simulink model "spike_detection"  (R2020a)
settings: Solver=FixedStepDiscrete  StartTime=0.0  StopTime=840000  RelTol=1e-3
libraries: hdlsllib x8, simulink x4
settings Model: FPTRunName=FPA_Reference  PacingRate=40  Creator=BuccelliLab  LastModifiedBy=diflo
settings SolverCC: AutoInsertRateTranBlk=on  MinimalZcImpactIntegration=on
settings DataIOCC: LimitDataPoints=on  SaveOutput=off  SaveTime=off  ReturnWorkspaceOutputs=off
settings OptimizationCC: BlockReduction=off  ConditionallyExecuteInputs=off  DefaultParameterBehavior=Inlined  LifeSpan=inf
settings DebuggingCC: SignalRangeChecking=warning  ReadBeforeWriteMsg=DisableAll  WriteAfterWriteMsg=DisableAll  WriteAfterReadMsg=DisableAll  AlgebraicLoopMsg=error  MultiTaskDSMMsg=none  SingleTaskRateTransMsg=error  ParameterDowncastMsg=warning  ParameterOverflowMsg=warning  AllowSymbolicDim=off  StrictBusMsg=ErrorOnBusTreatedAsVector  SFUnexpectedBacktrackingDiag=warning  SFNoUnconditionalDefaultTransitionDiag=warning  SFExecutionAtInitializationDiag=none  ArithmeticOperatorsInVariantConditions=warning
settings HardwareCC: ProdBitPerPointer=32  ProdBitPerSizeT=32  ProdBitPerPtrDiffT=32  ProdLargestAtomicFloat=None  ProdIntDivRoundTo=Undefined  ProdEndianess=Unspecified  ProdWordSize=32  ProdHWDeviceType=ASIC/FPGA->ASIC/FPGA  TargetBitPerPointer=64  TargetBitPerSizeT=64  TargetBitPerPtrDiffT=64  TargetLongLongMode=on  TargetIntDivRoundTo=Zero  TargetEndianess=LittleEndian  TargetWordSize=64  TargetHWDeviceType=Custom Processor->MATLAB Host Computer  ProdEqTarget=off
settings ModelReferenceCC: UpdateModelReferenceTargets=IfOutOfDate
settings SFSimCC: SFSimEcho=off  SimUseLocalCustomCode=off  CustomCodeUndefinedFunction=UseInterfaceOnly
settings RTWCC: RTWUseLocalCustomCode=off
settings CodeAppCC: StateflowObjectComments=on
settings GRTTargetCC: TargetLangStandard=C89/C90 (ANSI)
settings ConfigComp: CovScope=ReferencedModels  CovMetricSettings=dw  CovHtmlReporting=on  CovSaveCumulativeToWorkspaceVar=on  CovSaveSingleToWorkspaceVar=on  CovExternalEMLEnable=off  CovSFcnEnable=off

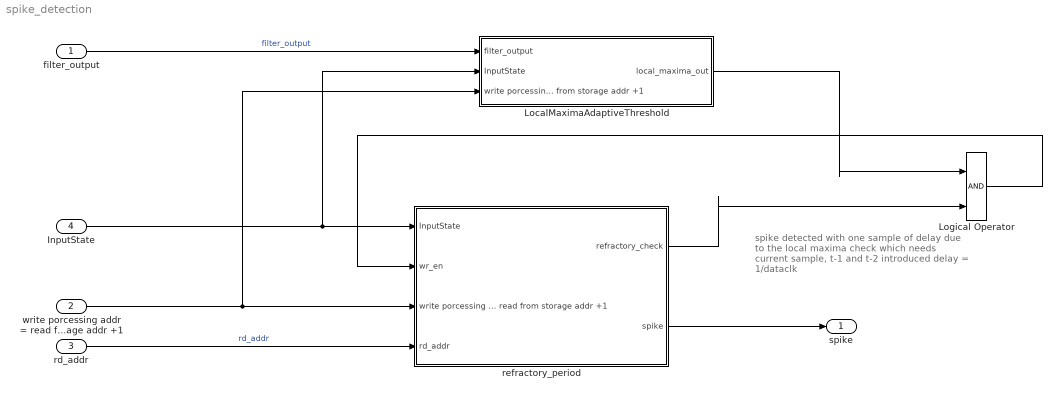
== system spike_detection ==
  note: spike detected with one sample of delay
      | due to the local maxima check which needs
      | current sample, t-1 and t-2
      |
      | introduced delay = 1/dataclk
  filter_output : Inport  OutDataTypeStr=uint16  PortDimensions=1  SampleTime=[1,0]
  write porcessing addr = read from storage addr +1 : Inport  Port=2  OutDataTypeStr=fixdt(0,9,0)  PortDimensions=1  SampleTime=[1,0]
  rd_addr : Inport  Port=3  OutDataTypeStr=fixdt(0,9,0)  PortDimensions=1  SampleTime=[1,0]
  InputState : Inport  Port=4  OutDataTypeStr=boolean  PortDimensions=1  SampleTime=[1,0]
  LocalMaximaAdaptiveThreshold : Subsystem
  Logical Operator : Logic  IconShape=distinctive  AllPortsSameDT=off  OutDataTypeStr=boolean
  refractory_period : Subsystem
  spike : Outport  OutDataTypeStr=uint16  PortDimensions=1  SampleTime=[1,0]
  wires:
  Logical Operator/1 -> refractory_period/2(wr_en)
  write porcessing addr = read from storage addr +1/1 -> refractory_period/3(write porcessing addr = read from storage addr +1), LocalMaximaAdaptiveThreshold/3(write porcessing addr = read from storage addr +1)
  rd_addr/1 -> refractory_period/4(rd_addr)  "rd_addr"
  refractory_period/2(spike) -> spike/1
  refractory_period/1(refractory_check) -> Logical Operator/2
  LocalMaximaAdaptiveThreshold/1(local_maxima_out) -> Logical Operator/1
  InputState/1 -> refractory_period/1(InputState), LocalMaximaAdaptiveThreshold/2(InputState)
  filter_output/1 -> LocalMaximaAdaptiveThreshold/1(filter_output)  "filter_output"

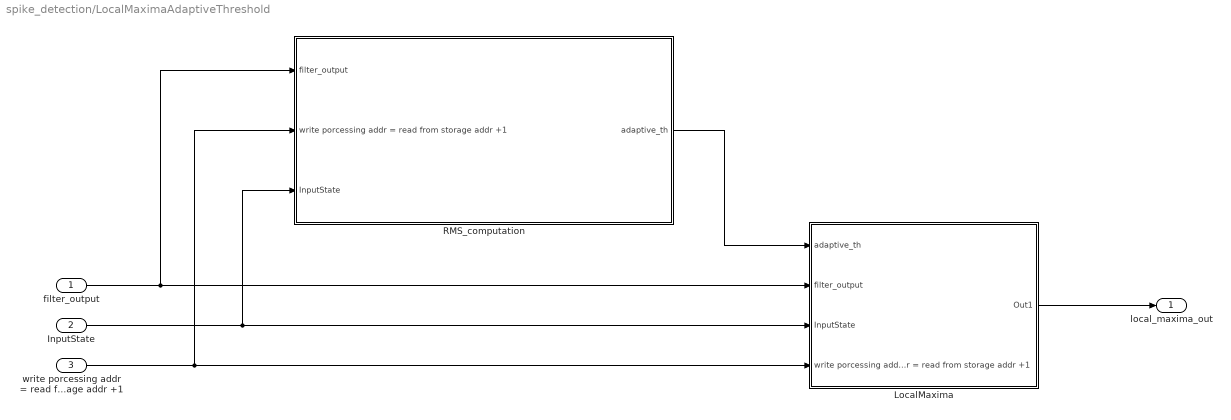
== system spike_detection/LocalMaximaAdaptiveThreshold ==
  filter_output : Inport
  InputState : Inport  Port=2
  write porcessing addr = read from storage addr +1 : Inport  Port=3
  LocalMaxima : Subsystem
  RMS_computation : Subsystem
  local_maxima_out : Outport
  wires:
  RMS_computation/1(adaptive_th) -> LocalMaxima/1(adaptive_th)
  LocalMaxima/1(Out1) -> local_maxima_out/1
  write porcessing addr = read from storage addr +1/1 -> LocalMaxima/4(write porcessing addr = read from storage addr +1), RMS_computation/2(write porcessing addr = read from storage addr +1)
  InputState/1 -> LocalMaxima/3(InputState), RMS_computation/3(InputState)
  filter_output/1 -> LocalMaxima/2(filter_output), RMS_computation/1(filter_output)

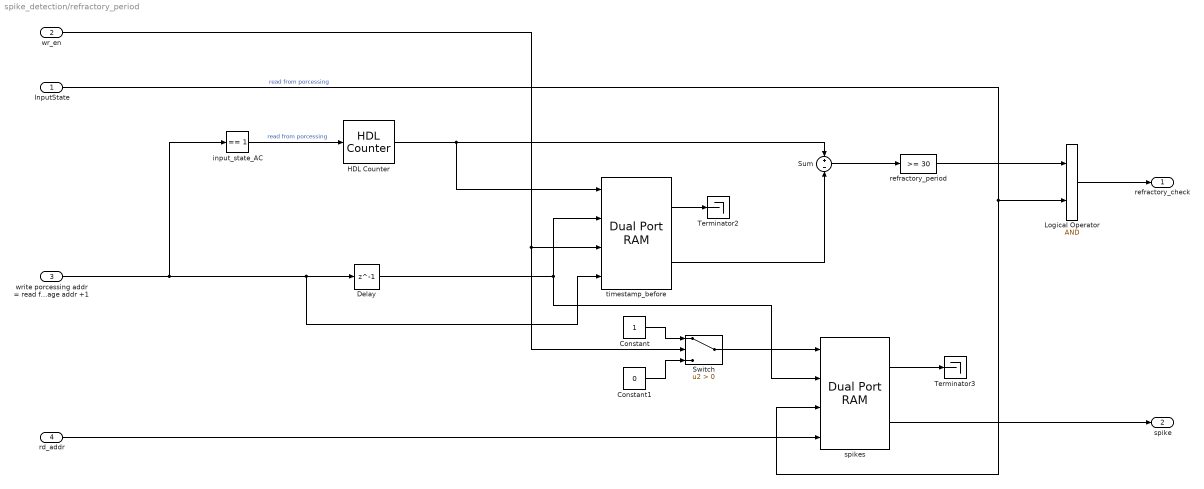
== system spike_detection/refractory_period ==
  InputState : Inport
  wr_en : Inport  Port=2
  write porcessing addr = read from storage addr +1 : Inport  Port=3
  rd_addr : Inport  Port=4
  Constant : Constant  OutDataTypeStr=uint16  SampleTime=-1
  Constant1 : Constant  Value=0  OutDataTypeStr=uint16  SampleTime=-1
  Delay : Delay  DelayLength=1  InitialCondition=0
  HDL Counter : hdlsllib/Sources/HDL Counter  CountType=Free running  CountInit=0  CountStep=1  CountMax=2^32  CountFromType=Initial value  CountFrom=0  CountResetPort=off  CountLoadPort=off  CountEnbPort=on  CountDirPort=off  CountDataType=Unsigned  CountWordLen=32  CountFracLen=0  CountSampTime=1
  Logical Operator : Logic  IconShape=distinctive  AllPortsSameDT=off  OutDataTypeStr=boolean
  Sum : Sum  Inputs=+-
  Switch : Switch  Criteria=u2 > Threshold
  Terminator2 : Terminator
  Terminator3 : Terminator
  input_state_AC : simulink/Logic and Bit Operations/Compare To Constant  relop===  const=1  OutDataTypeStr=boolean
  refractory_period : simulink/Logic and Bit Operations/Compare To Constant  relop=>=  const=30  OutDataTypeStr=boolean
  spikes : hdlsllib/HDL RAMs/Dual Port RAM  ram_size=9
      settings: SourceProductBaseCode=SL
  timestamp_before : hdlsllib/HDL RAMs/Dual Port RAM  ram_size=9
      settings: SourceProductBaseCode=SL
  refractory_check : Outport
  spike : Outport  Port=2
  wires:
  Constant1/1 -> Switch/3
  Switch/1 -> spikes/1
  Constant/1 -> Switch/1
  HDL Counter/1 -> Sum/1, timestamp_before/1
  input_state_AC/1 -> HDL Counter/1  "read from porcessing"
  Logical Operator/1 -> refractory_check/1
  refractory_period/1 -> Logical Operator/1
  InputState/1 -> Logical Operator/2, spikes/3  "read from porcessing"
  Sum/1 -> refractory_period/1
  spikes/1 -> Terminator3/1
  rd_addr/1 -> spikes/4
  timestamp_before/2 -> Sum/2
  wr_en/1 -> timestamp_before/3, Switch/2
  write porcessing addr = read from storage addr +1/1 -> timestamp_before/4, Delay/1, input_state_AC/1
  spikes/2 -> spike/1
  Delay/1 -> timestamp_before/2, spikes/2
  timestamp_before/1 -> Terminator2/1

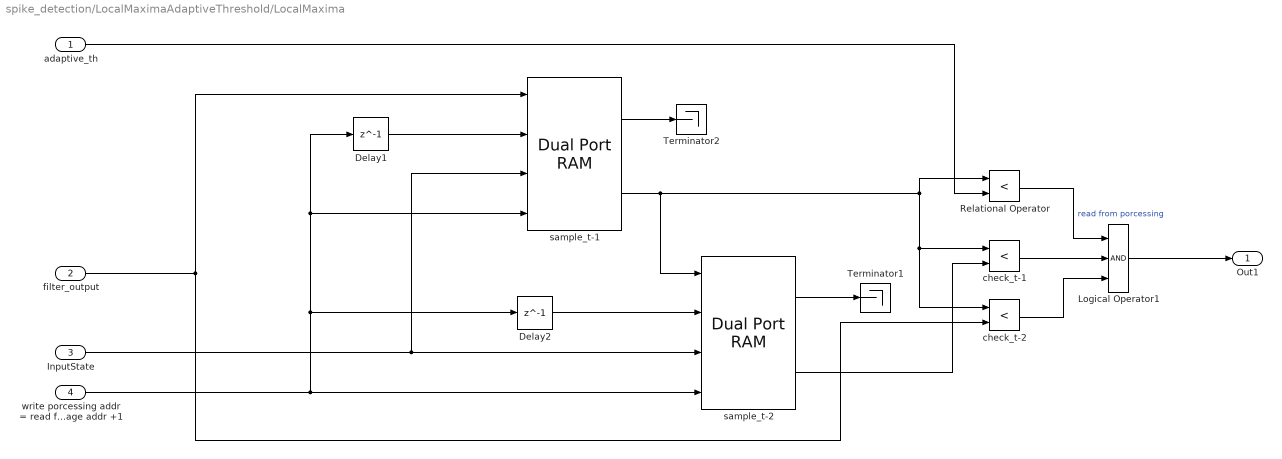
== system spike_detection/LocalMaximaAdaptiveThreshold/LocalMaxima ==
  adaptive_th : Inport
  filter_output : Inport  Port=2
  InputState : Inport  Port=3
  write porcessing addr = read from storage addr +1 : Inport  Port=4
  Delay1 : Delay  DelayLength=1  InitialCondition=0
  Delay2 : Delay  DelayLength=1  InitialCondition=0
  Logical Operator1 : Logic  Inputs=3  IconShape=distinctive  AllPortsSameDT=off  OutDataTypeStr=boolean
  Relational Operator : RelationalOperator  Operator=<  OutDataTypeStr=boolean  RndMeth=Simplest
  Terminator1 : Terminator
  Terminator2 : Terminator
  check_t-1 : RelationalOperator  Operator=<  OutDataTypeStr=boolean  RndMeth=Simplest
  check_t-2 : RelationalOperator  Operator=<  OutDataTypeStr=boolean  RndMeth=Simplest
  sample_t-1 : hdlsllib/HDL RAMs/Dual Port RAM  ram_size=9
      settings: SourceProductBaseCode=SL
  sample_t-2 : hdlsllib/HDL RAMs/Dual Port RAM  ram_size=9
      settings: SourceProductBaseCode=SL
  Out1 : Outport
  wires:
  adaptive_th/1 -> Relational Operator/2
  Logical Operator1/1 -> Out1/1
  InputState/1 -> sample_t-1/3, sample_t-2/3
  Delay2/1 -> sample_t-2/2
  check_t-1/1 -> Logical Operator1/2
  sample_t-2/1 -> Terminator1/1
  write porcessing addr = read from storage addr +1/1 -> sample_t-1/4, Delay1/1, Delay2/1, sample_t-2/4
  sample_t-1/1 -> Terminator2/1
  filter_output/1 -> check_t-2/2, sample_t-1/1
  sample_t-2/2 -> check_t-1/2
  check_t-2/1 -> Logical Operator1/3
  sample_t-1/2 -> check_t-1/1, check_t-2/1, Relational Operator/1, sample_t-2/1
  Relational Operator/1 -> Logical Operator1/1  "read from porcessing"
  Delay1/1 -> sample_t-1/2

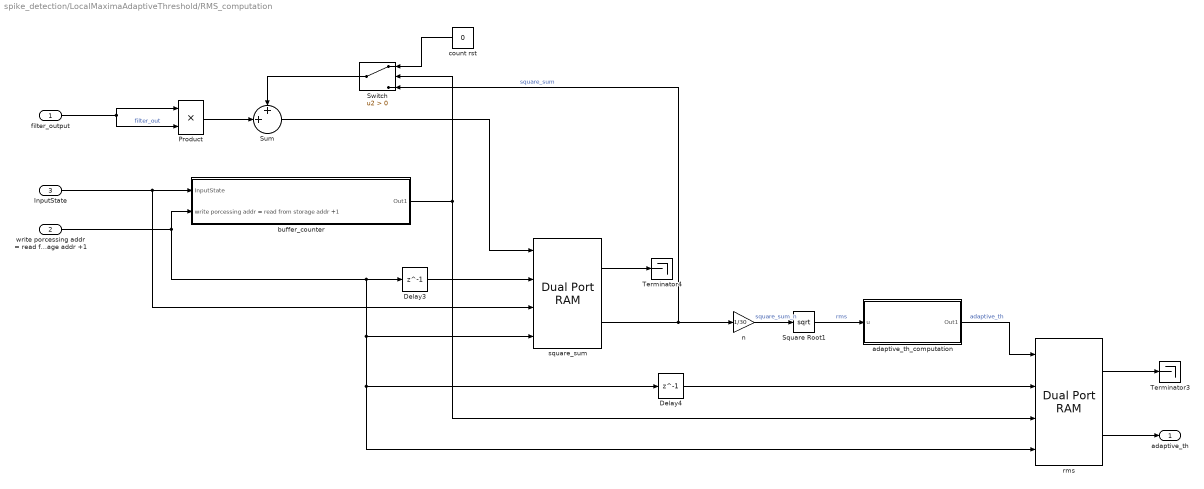
== system spike_detection/LocalMaximaAdaptiveThreshold/RMS_computation ==
  filter_output : Inport
  write porcessing addr = read from storage addr +1 : Inport  Port=2
  InputState : Inport  Port=3
  Delay3 : Delay  DelayLength=1  InitialCondition=0
  Delay4 : Delay  DelayLength=1  InitialCondition=0
  Product : Product
  Square Root1 : Sqrt  OutDataTypeStr=uint16  SaturateOnIntegerOverflow=on
  Sum : Sum  Inputs=++|  OutDataTypeStr=uint64
  Switch : Switch  Criteria=u2 > Threshold  OutDataTypeStr=uint64
  Terminator3 : Terminator
  Terminator4 : Terminator
  adaptive_th_computation : Subsystem
  buffer_counter : Subsystem
  count rst : Constant  Value=0  OutDataTypeStr=uint64  SampleTime=-1
  n : Gain  Gain=1/30  OutDataTypeStr=fixdt(0,40,0)
  rms : hdlsllib/HDL RAMs/Dual Port RAM  ram_size=9
      settings: SourceProductBaseCode=SL
  square_sum : hdlsllib/HDL RAMs/Dual Port RAM  ram_size=9
      settings: SourceProductBaseCode=SL
  adaptive_th : Outport
  wires:
  adaptive_th_computation/1(Out1) -> rms/1  "adaptive_th"
  Square Root1/1 -> adaptive_th_computation/1(u)  "rms"
  rms/2 -> adaptive_th/1
  filter_output/1 -> Product/1, Product/2  "filter_out"
  InputState/1 -> buffer_counter/1(InputState), square_sum/3
  square_sum/1 -> Terminator4/1
  Delay3/1 -> square_sum/2
  Switch/1 -> Sum/1
  Delay4/1 -> rms/2
  Product/1 -> Sum/2
  rms/1 -> Terminator3/1
  buffer_counter/1(Out1) -> Switch/2, rms/3
  Sum/1 -> square_sum/1
  square_sum/2 -> Switch/3, n/1  "square_sum"
  count rst/1 -> Switch/1
  write porcessing addr = read from storage addr +1/1 -> Delay3/1, square_sum/4, Delay4/1, rms/4, buffer_counter/2(write porcessing addr = read from storage addr +1)
  n/1 -> Square Root1/1  "square_sum_n"

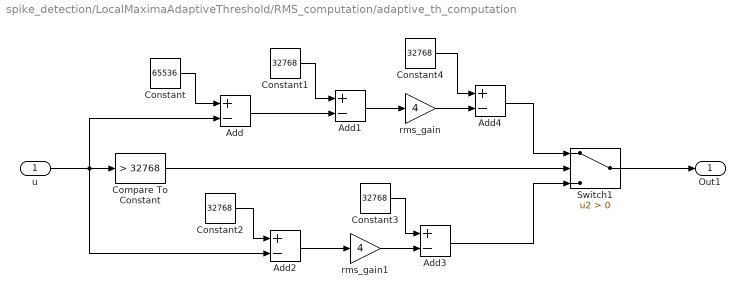
== system spike_detection/LocalMaximaAdaptiveThreshold/RMS_computation/adaptive_th_computation ==
  u : Inport
  Add{,1..4} (5 alike) : Sum  Inputs=+-  OutDataTypeStr=uint16
  Compare To Constant : simulink/Logic and Bit Operations/Compare To Constant  relop=>  const=32768  OutDataTypeStr=boolean
  Constant : Constant  Value=65536  OutDataTypeStr=uint16  SampleTime=-1
  Constant{1..4} (4 alike) : Constant  Value=32768  OutDataTypeStr=uint16  SampleTime=-1
  Switch1 : Switch  Criteria=u2 > Threshold
  rms_gain : Gain  Gain=4  OutDataTypeStr=uint16
  rms_gain1 : Gain  Gain=4  OutDataTypeStr=uint16
  Out1 : Outport
  wires:
  Switch1/1 -> Out1/1
  u/1 -> Compare To Constant/1, Add/2, Add2/2
  Add1/1 -> rms_gain/1
  Add2/1 -> rms_gain1/1
  Constant3/1 -> Add3/1
  rms_gain1/1 -> Add3/2
  Add4/1 -> Switch1/1
  Constant1/1 -> Add1/1
  rms_gain/1 -> Add4/2
  Constant4/1 -> Add4/1
  Add/1 -> Add1/2
  Compare To Constant/1 -> Switch1/2
  Constant/1 -> Add/1
  Constant2/1 -> Add2/1
  Add3/1 -> Switch1/3

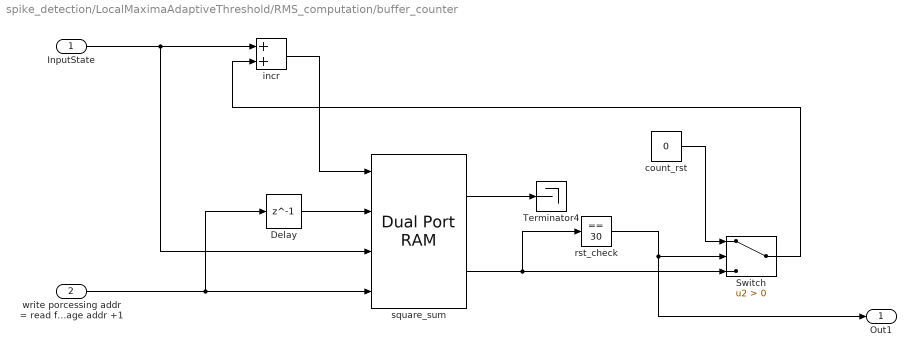
== system spike_detection/LocalMaximaAdaptiveThreshold/RMS_computation/buffer_counter ==
  InputState : Inport
  write porcessing addr = read from storage addr +1 : Inport  Port=2
  Delay : Delay  DelayLength=1  InitialCondition=0
  Switch : Switch  Criteria=u2 > Threshold  OutDataTypeStr=uint32
  Terminator4 : Terminator
  count_rst : Constant  Value=0  OutDataTypeStr=uint16  SampleTime=-1
  incr : Sum  AccumDataTypeStr=uint32
  rst_check : simulink/Logic and Bit Operations/Compare To Constant  relop===  const=30  OutDataTypeStr=boolean
  square_sum : hdlsllib/HDL RAMs/Dual Port RAM  ram_size=9
      settings: SourceProductBaseCode=SL
  Out1 : Outport
  wires:
  rst_check/1 -> Switch/2, Out1/1
  write porcessing addr = read from storage addr +1/1 -> Delay/1, square_sum/4
  Switch/1 -> incr/2
  InputState/1 -> square_sum/3, incr/1
  incr/1 -> square_sum/1
  Delay/1 -> square_sum/2
  count_rst/1 -> Switch/1
  square_sum/1 -> Terminator4/1
  square_sum/2 -> Switch/3, rst_check/1
